simulink library "ctd"  (Simulink 8.1)
settings: Solver=ode1  StartTime=0.0  StopTime=Inf  FixedStep=0.001  RelTol=1e-3
PostLoadFcn:
  | , if any(exist('dsrtsu_mdlpostloadfcn', 'file') == [2, 3, 6]), try dsrtsu_mdlpostloadfcn('Execute', bdroot); catch fprintf('Error in PostLoadFcn (dsrtsu_mdlpostloadfcn) for model "%s":\n %s\n', bdroot, lasterr); end, end,
undefined symbols (not defined in the file or in its folder): KACC_TransDistControlPTCMargin_m, KACC_TransDistControlPTCPerc_perc, KACC_TransDistCtrlPTCFixedMarg_flg
settings Model: DSRTSU_INTERNAL_RTI_VER=450  DSRTSU_INTERNAL_RTI_TYPE=rti1401  RTICANMMDATA=struct('GeneralSetupData',struct('modelroot','C:\Users\idiada\Desktop\HAITEC_Taiwan\trunk\AdasDragon\software\sw_development\arch\app\acc','generalsettings',struct('filesettings',struct('destfolder',struct('Name','RTICANMM_FILES','Check',1),'buildfolder',struct('Name','.','Check',1),'AbsDestfolder',struct('Name','C:\Users\idiada\Desktop\HAITEC_Taiwan\trunk\AdasDragon\software\sw_development\arch\app\acc\RTICANMM_FILES'),'AbsBuildfolder',struct('Name','C:\Users\idiada\Desktop\HAITEC_Taiwan\trunk\AdasDragon\software\sw_development\arch\app\acc'))),'options',struct('addpaths',1,'rmpaths',1,'addtrcexclusion',logical(1),'cannavigator',struct('checkmonitoring',0),'show_usrtrc',0,'use_usrtrc',0),'advanced',struct('options',[1 1 1 1 1 1 1 1 1 1 1 1 1 1 1 1 1 1 1 1 1 1 1 1 1 1 1 1 1 1 1 1 1 1 1 1 1 1 1 1 1 1 1 1 1 1 1 1 1 1 1 1 1 1 1 1 1 1 1 1 1 1 1 1 1 1 1 1 1 1 1 1 1 1 1 1 1 1 1 1 1 1 1 1 1 1 1 1 1 1 1 1 1 1 1 1 1 1 1 1]),'MPSetup',{{}},'modelname','ctd','block','ctd'))  DSRTSU_INTERNAL_RTIFPGA=40  Creator=idiada  LastModifiedBy=idiada

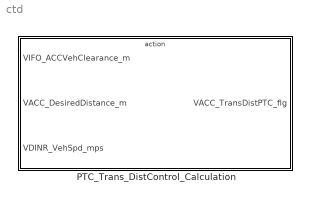
== system ctd ==
  PTC_Trans_DistControl_Calculation : Subsystem  TreatAsAtomicUnit=on

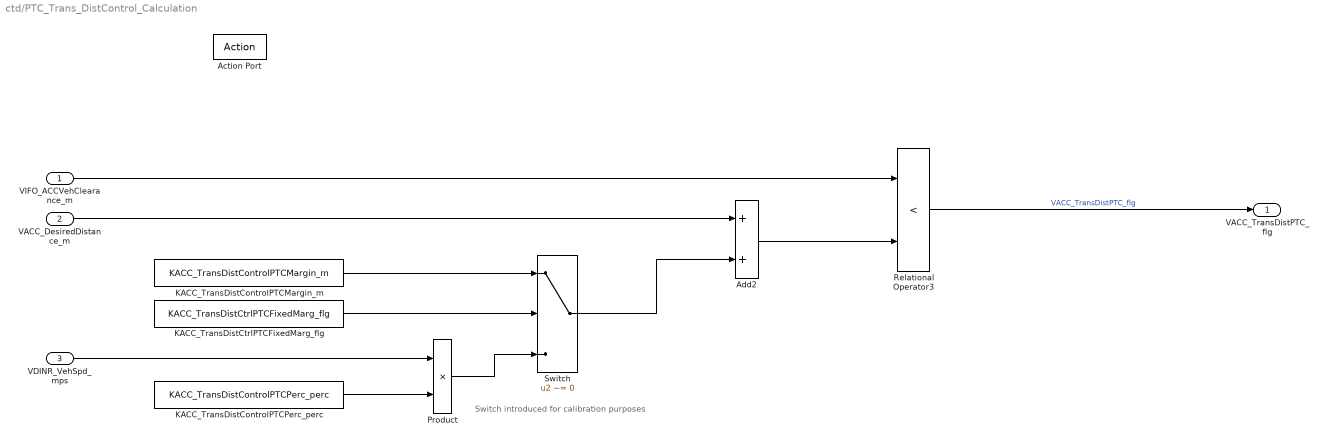
== system ctd/PTC_Trans_DistControl_Calculation ==
  note: Switch introduced for calibration purposes
  VIFO_ACCVehClearance_m : Inport
  VACC_DesiredDistance_m : Inport  Port=2
  VDINR_VehSpd_mps : Inport  Port=3
  Action Port : ActionPort
  Add2 : Sum
  KACC_TransDistControlPTCMargin_m : Constant  Value=KACC_TransDistControlPTCMargin_m
  KACC_TransDistControlPTCPerc_perc : Constant  Value=KACC_TransDistControlPTCPerc_perc
  KACC_TransDistCtrlPTCFixedMarg_flg : Constant  Value=KACC_TransDistCtrlPTCFixedMarg_flg
  Product : Product
  Relational Operator3 : RelationalOperator  Operator=<  OutDataTypeStr=boolean
  Switch : Switch  Criteria=u2 ~= 0
  VACC_TransDistPTC_flg : Outport
  wires:
  Switch/1 -> Add2/2
  KACC_TransDistControlPTCMargin_m/1 -> Switch/1
  VDINR_VehSpd_mps/1 -> Product/1
  KACC_TransDistCtrlPTCFixedMarg_flg/1 -> Switch/2
  KACC_TransDistControlPTCPerc_perc/1 -> Product/2
  Product/1 -> Switch/3
  Relational Operator3/1 -> VACC_TransDistPTC_flg/1  "VACC_TransDistPTC_flg"
  Add2/1 -> Relational Operator3/2
  VIFO_ACCVehClearance_m/1 -> Relational Operator3/1
  VACC_DesiredDistance_m/1 -> Add2/1
